simulink model "cleanmodel"  (R2024a)
settings: Solver=VariableStepAuto  StartTime=0.0  StopTime=50  RelTol=1e-3
values from neighbouring files (symbols this model uses):
  b = 1    [Hydrone_model_code.m]
  L = 1.16    [Hydrone_model_code.m]
  r = 1    [Hydrone_model_code.m]
  w = .7    (= 0.7)    [Hydrone_model_code.m]
  WGS1984 = [ 0 0 0; 10 0 0; 10 10 0; 11 20 0; 20 20 0]    [Hydrone_model_code.m]    (also in coverageroi.m = WGS1984(1:size(WGS1984,1)-1,:))
libraries: slpidlib x2, shared6dof x1, robotcorelib x1, uavutilslib x1, uavalgslib x1
settings Model: PacingRate=18  Creator=awolek  LastModifiedBy=alexn
settings RTWCC: GPUComputeCapability=3.5

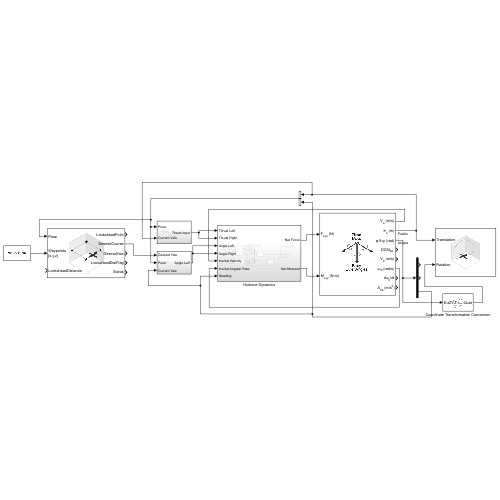
[thumbnail: Simulink's stored preview of the top-level diagram]
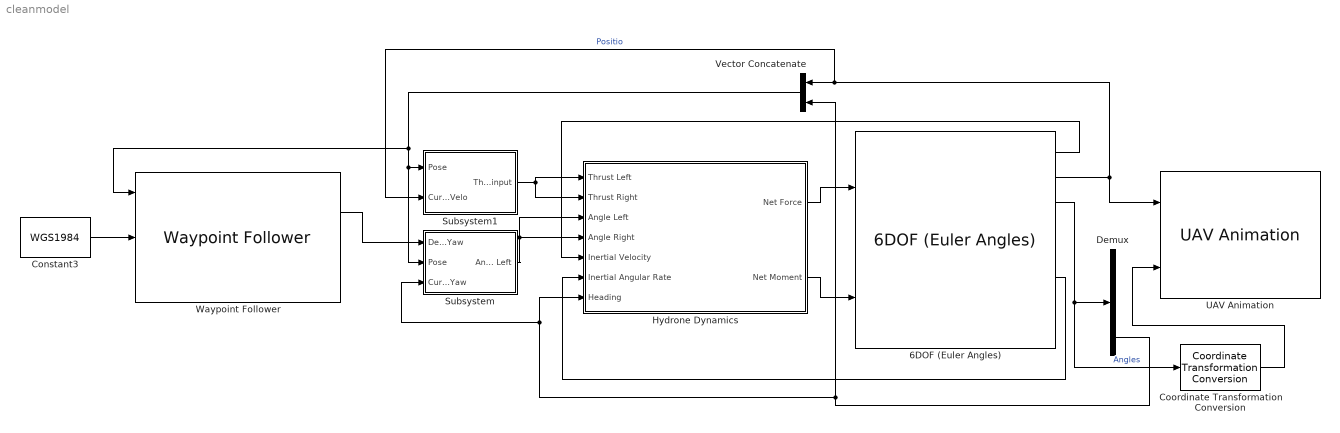
== system cleanmodel ==
  6DOF (Euler Angles) : shared6dof/6DOF (Euler Angles)  units=Metric (MKS)  mtype=Fixed  rep=Euler Angles  xme_0=[0 0 0]  Vm_0=[0 0 0]  eul_0=[0 0 0]  pm_0=[0 0 0]  mass_0=m  mass_e=0.5  mass_f=2.0  inertia=i  inertia_e=eye(3)  inertia_f=2*eye(3)  k_quat=1.0  vre_flag=on  abi_flag=off  aMode=0  xme_statename=''  Vm_statename=''  eul_statename=''  quat_statename=''  pm_statename=''  mass_statename=''
  Constant3 : Constant  Value=WGS1984
  Coordinate Transformation Conversion : robotcorelib/Coordinate Transformation Conversion  InputRepresentation=Euler Angles  InputEulerSequence=ZYZ  ShowTrVecInputPort=on  OutputRepresentation=Quaternion  OutputEulerSequence=ZYX  ShowTrVecOutputPort=on  SimulateUsing=Interpreted execution
      settings: LibrarySourceBlock=uavutilslib/Coordinate Transformation Conversion
  Demux : Demux  Outputs=3
  Hydrone Dynamics : Subsystem
  Subsystem : Subsystem
  Subsystem1 : Subsystem
  UAV Animation : uavutilslib/UAV Animation  UAVType=FixedWing  UAVSize=1  InertialZDirection=Down  SampleTime=-1
  Vector Concatenate : Concatenate
  Waypoint Follower : uavalgslib/Waypoint Follower  UAVType=fixed-wing  StartFrom=first  TransitionRadiusSource=internal  TransitionRadius=1  MinLookaheadDistance=1  YawInput=off  ShowCrossTrackErrorOutput=off  ShowStatusOutput=on  SimulateUsing=Interpreted execution
  wires:
  6DOF (Euler Angles)/2 -> UAV Animation/1, Subsystem1/2(Current Velo), Vector Concatenate/1  "Positio"
  Hydrone Dynamics/1(Net Force) -> 6DOF (Euler Angles)/1
  Hydrone Dynamics/2(Net Moment) -> 6DOF (Euler Angles)/2
  6DOF (Euler Angles)/3 -> Coordinate Transformation Conversion/1, Demux/1  "Angles"
  6DOF (Euler Angles)/6 -> Hydrone Dynamics/6(Inertial Angular Rate)
  Coordinate Transformation Conversion/1 -> UAV Animation/2
  Constant3/1 -> Waypoint Follower/2
  Vector Concatenate/1 -> Subsystem/2(Pose), Subsystem1/1(Pose), Waypoint Follower/1
  6DOF (Euler Angles)/1 -> Hydrone Dynamics/5(Inertial Velocity)
  Waypoint Follower/2 -> Subsystem/1(Desired Yaw)
  Subsystem/1(Angle Left) -> Hydrone Dynamics/3(Angle Left), Hydrone Dynamics/4(Angle Right)
  Demux/3 -> Subsystem/3(Current Yaw), Hydrone Dynamics/7(Heading), Vector Concatenate/2
  Subsystem1/1(Thrust input) -> Hydrone Dynamics/1(Thrust Left), Hydrone Dynamics/2(Thrust Right)

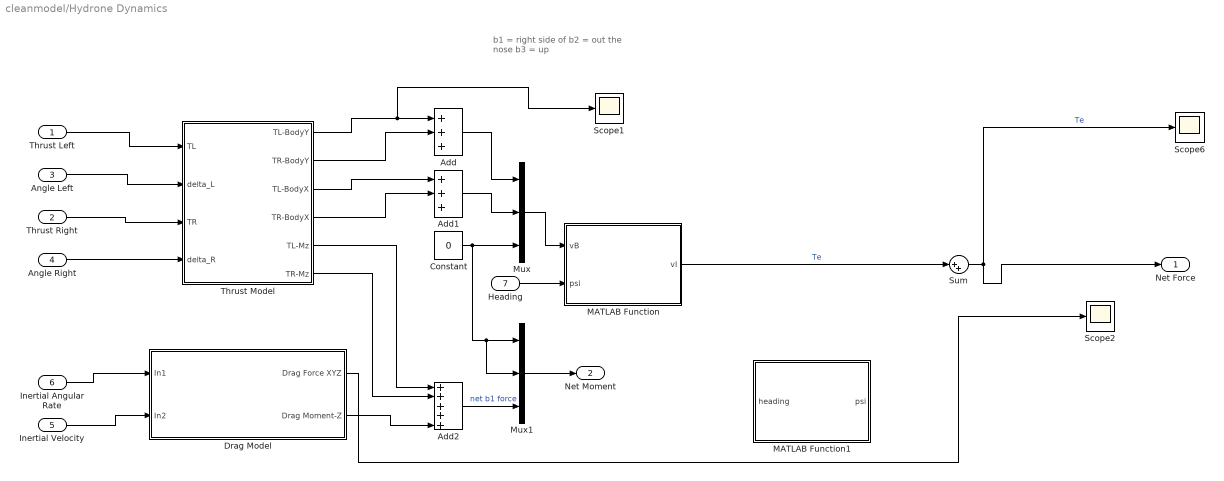
== system cleanmodel/Hydrone Dynamics ==
  note: b1 = right side of
      | b2 = out the nose
      | b3 = up
  Thrust Left : Inport
  Thrust Right : Inport  Port=2
  Angle Left : Inport  Port=3
  Angle Right : Inport  Port=4
  Inertial Velocity : Inport  Port=5
  Inertial Angular Rate : Inport  Port=6
  Heading : Inport  Port=7
  Add : Sum  Inputs=+++
  Add1 : Sum  Inputs=+++
  Add2 : Sum  Inputs=+++++
  Constant : Constant  Value=0
  Drag Model : Subsystem
  MATLAB Function : MATLAB Function  TreatAsAtomicUnit=on
  MATLAB Function1 : MATLAB Function  TreatAsAtomicUnit=on
  Mux : Mux  Inputs=3
  Mux1 : Mux  Inputs=3
  Scope1 : Scope
  Scope2 : Scope
  Scope6 : Scope
  Sum : Sum  Inputs=|++
  Thrust Model : Subsystem
  Net Force : Outport
  Net Moment : Outport  Port=2
  wires:
  Add2/1 -> Mux1/3  "net b1 force"
  Constant/1 -> Mux/3, Mux1/2, Mux1/1
  Drag Model/2(Drag Moment-Z) -> Add2/5
  Mux1/1 -> Net Moment/1
  Thrust Right/1 -> Thrust Model/3(TR)
  Angle Right/1 -> Thrust Model/4(delta_R)
  Inertial Angular Rate/1 -> Drag Model/1(In1)
  Thrust Model/6(TR-Mz) -> Add2/2
  Thrust Model/1(TL-BodyY) -> Scope1/1, Add/1
  Thrust Model/2(TR-BodyY) -> Add/2
  Inertial Velocity/1 -> Drag Model/2(In2)
  Thrust Model/3(TL-BodyX) -> Add1/1
  Angle Left/1 -> Thrust Model/2(delta_L)
  Thrust Model/5(TL-Mz) -> Add2/1
  Thrust Left/1 -> Thrust Model/1(TL)
  Thrust Model/4(TR-BodyX) -> Add1/2
  Add/1 -> Mux/1
  Add1/1 -> Mux/2
  Sum/1 -> Net Force/1, Scope6/1  "Te"
  Heading/1 -> MATLAB Function/2(psi)
  MATLAB Function/1(vI) -> Sum/1  "Te"
  Drag Model/1(Drag Force XYZ) -> Scope2/1
  Mux/1 -> MATLAB Function/1(vB)

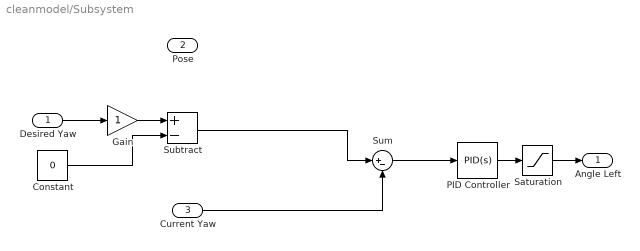
== system cleanmodel/Subsystem ==
  Desired Yaw : Inport
  Pose : Inport  Port=2
  Current Yaw : Inport  Port=3
  Constant : Constant  Value=0
  Gain : Gain
  PID Controller : slpidlib/PID Controller  Controller=PID  Form=Parallel  TimeDomain=Continuous-time  UseExternalTs=off  SampleTime=-1  IntegratorMethod=Forward Euler  FilterMethod=Forward Euler  ControllerParametersSource=internal  P=1  I=.01  UseKiTs=off  D=.001  UseExternalDerivativeSource=off  N=100  UseFilter=on  TunerSelectOption=Transfer Function Based (PID Tuner App)  InitialConditionSource=internal  InitialConditionForIntegrator=0  InitialConditionForFilter=0  DifferentiatorICPrevScaledInput=0  ExternalReset=none  TrackingMode=off  Kt=1  LimitOutput=off  SatLimitsSource=internal  UpperSaturationLimit=inf  LowerSaturationLimit=-inf  LinearizeAsGain=on  AntiWindupMode=none  Kb=1  LimitIntegrator=off  UpperIntegratorSaturationLimit=inf  LowerIntegratorSaturationLimit=-inf  POutMin=[]  POutMax=[]  IOutMin=[]  IOutMax=[]  DOutMin=[]  DOutMax=[]  NOutMin=[]  NOutMax=[]  SumOutMin=[]  SumOutMax=[]  SaturationOutMin=[]  SaturationOutMax=[]  PParamMin=[]  PParamMax=[]  IParamMin=[]  IParamMax=[]  DParamMin=[]  DParamMax=[]  NParamMin=[]  NParamMax=[]  KbParamMin=[]  KbParamMax=[]  KtParamMin=[]  KtParamMax=[]  KbOutMin=[]  KbOutMax=[]  KtOutMin=[]  KtOutMax=[]  IntegratorOutMin=[]  IntegratorOutMax=[]  FilterOutMin=[]  FilterOutMax=[]  SumI1OutMin=[]  SumI1OutMax=[]  SumI2OutMin=[]  SumI2OutMax=[]  SumI3OutMin=[]  SumI3OutMax=[]  SumI4OutMin=[]  SumI4OutMax=[]  SumDOutMin=[]  SumDOutMax=[]  DifferentiatorOutMin=[]  DifferentiatorOutMax=[]  FilterDiffOutCoefMin=[]  FilterDiffOutCoefMax=[]  ReciprocalOutMin=[]  ReciprocalOutMax=[]  SumDenOutMin=[]  SumDenOutMax=[]  SumNumOutMin=[]  SumNumOutMax=[]  DivideOutMin=[]  DivideOutMax=[]  UdiffTsProdOutMin=[]  UdiffTsProdOutMax=[]  NTsProdOutMin=[]  NTsProdOutMax=[]  UintegralTsProdOutMin=[]  UintegralTsProdOutMax=[]  UngainTsProdOutMin=[]  UngainTsProdOutMax=[]  ClampingZeroOutDataTypeStr=Inherit: Inherit via back propagation  ClampingZeroOutMin=[]  ClampingZeroOutMax=[]  FilterDenConstantOutDataTypeStr=Inherit: Inherit via back propagation  FilterDenConstantOutMin=[]  FilterDenConstantOutMax=[]  PCopyOutDataTypeStr=Inherit: Inherit via back propagation  PCopyOutMin=[]  PCopyOutMax=[]  NCopyOutDataTypeStr=Inherit: Inherit via back propagation  NCopyOutMin=[]  NCopyOutMax=[]  IntegratorContinuousStateAttributes=''  IntegratorStateMustResolveToSignalObject=off  IntegratorRTWStateStorageClass=Auto  FilterContinuousStateAttributes=''  FilterStateMustResolveToSignalObject=off  FilterRTWStateStorageClass=Auto  ParallelPVariant=InternalParameters  IdealPVariant=Disabled  IVariant=InternalParameters  DVariant=InternalParameters  IntegratorVariant=Continuous  SatVariant=Disabled  AWVariant=Passthrough  PCopyVariant=Disabled  TRVariant=Disabled  FdbkBlocksVariant=Forward  IdealPFdbkVariant=Disabled  SatFdbkVariant=Disabled  DerivativeFilterVariant=ContFilter  NVariant=InternalParameters  NCopyVariant=Disabled  FilterICVariant=InternalICsFilter  IntegratorICVariant=InternalICs  ExternalResetVariant=Disabled  TRSumVariant=Passthrough  SumFdbkVariant=Disabled  SumVariant=Sum_PID  TsampFilterVariant=InternalTs  TsampNgainVariant=Passthrough  TsampIntegralVariant=Disabled_SignalSpec  ExternalSaturationOutDataTypeStr=Inherit: Same as second input  DerivativeSourceVariant=ErrorSignal
  Saturation : Saturate  UpperLimit=0.78  LowerLimit=-0.78
  Subtract : Sum  Inputs=+-
  Sum : Sum  Inputs=|+-
  Angle Left : Outport
  wires:
  PID Controller/1 -> Saturation/1
  Sum/1 -> PID Controller/1
  Current Yaw/1 -> Sum/2
  Desired Yaw/1 -> Gain/1
  Gain/1 -> Subtract/1
  Constant/1 -> Subtract/2
  Subtract/1 -> Sum/1
  Saturation/1 -> Angle Left/1

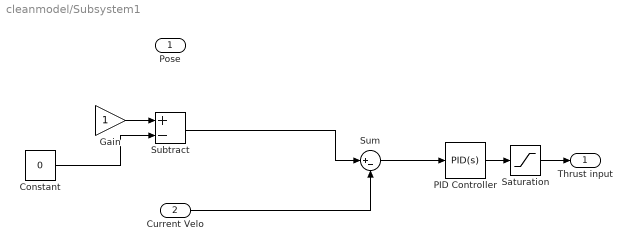
== system cleanmodel/Subsystem1 ==
  Pose : Inport
  Current Velo : Inport  Port=2
  Constant : Constant  Value=0
  Gain : Gain
  PID Controller : slpidlib/PID Controller  Controller=PID  Form=Parallel  TimeDomain=Continuous-time  UseExternalTs=off  SampleTime=-1  IntegratorMethod=Forward Euler  FilterMethod=Forward Euler  ControllerParametersSource=internal  P=1  I=.01  UseKiTs=off  D=.001  UseExternalDerivativeSource=off  N=100  UseFilter=on  TunerSelectOption=Transfer Function Based (PID Tuner App)  InitialConditionSource=internal  InitialConditionForIntegrator=0  InitialConditionForFilter=0  DifferentiatorICPrevScaledInput=0  ExternalReset=none  TrackingMode=off  Kt=1  LimitOutput=off  SatLimitsSource=internal  UpperSaturationLimit=inf  LowerSaturationLimit=-inf  LinearizeAsGain=on  AntiWindupMode=none  Kb=1  LimitIntegrator=off  UpperIntegratorSaturationLimit=inf  LowerIntegratorSaturationLimit=-inf  POutMin=[]  POutMax=[]  IOutMin=[]  IOutMax=[]  DOutMin=[]  DOutMax=[]  NOutMin=[]  NOutMax=[]  SumOutMin=[]  SumOutMax=[]  SaturationOutMin=[]  SaturationOutMax=[]  PParamMin=[]  PParamMax=[]  IParamMin=[]  IParamMax=[]  DParamMin=[]  DParamMax=[]  NParamMin=[]  NParamMax=[]  KbParamMin=[]  KbParamMax=[]  KtParamMin=[]  KtParamMax=[]  KbOutMin=[]  KbOutMax=[]  KtOutMin=[]  KtOutMax=[]  IntegratorOutMin=[]  IntegratorOutMax=[]  FilterOutMin=[]  FilterOutMax=[]  SumI1OutMin=[]  SumI1OutMax=[]  SumI2OutMin=[]  SumI2OutMax=[]  SumI3OutMin=[]  SumI3OutMax=[]  SumI4OutMin=[]  SumI4OutMax=[]  SumDOutMin=[]  SumDOutMax=[]  DifferentiatorOutMin=[]  DifferentiatorOutMax=[]  FilterDiffOutCoefMin=[]  FilterDiffOutCoefMax=[]  ReciprocalOutMin=[]  ReciprocalOutMax=[]  SumDenOutMin=[]  SumDenOutMax=[]  SumNumOutMin=[]  SumNumOutMax=[]  DivideOutMin=[]  DivideOutMax=[]  UdiffTsProdOutMin=[]  UdiffTsProdOutMax=[]  NTsProdOutMin=[]  NTsProdOutMax=[]  UintegralTsProdOutMin=[]  UintegralTsProdOutMax=[]  UngainTsProdOutMin=[]  UngainTsProdOutMax=[]  ClampingZeroOutDataTypeStr=Inherit: Inherit via back propagation  ClampingZeroOutMin=[]  ClampingZeroOutMax=[]  FilterDenConstantOutDataTypeStr=Inherit: Inherit via back propagation  FilterDenConstantOutMin=[]  FilterDenConstantOutMax=[]  PCopyOutDataTypeStr=Inherit: Inherit via back propagation  PCopyOutMin=[]  PCopyOutMax=[]  NCopyOutDataTypeStr=Inherit: Inherit via back propagation  NCopyOutMin=[]  NCopyOutMax=[]  IntegratorContinuousStateAttributes=''  IntegratorStateMustResolveToSignalObject=off  IntegratorRTWStateStorageClass=Auto  FilterContinuousStateAttributes=''  FilterStateMustResolveToSignalObject=off  FilterRTWStateStorageClass=Auto  ParallelPVariant=InternalParameters  IdealPVariant=Disabled  IVariant=InternalParameters  DVariant=InternalParameters  IntegratorVariant=Continuous  SatVariant=Disabled  AWVariant=Passthrough  PCopyVariant=Disabled  TRVariant=Disabled  FdbkBlocksVariant=Forward  IdealPFdbkVariant=Disabled  SatFdbkVariant=Disabled  DerivativeFilterVariant=ContFilter  NVariant=InternalParameters  NCopyVariant=Disabled  FilterICVariant=InternalICsFilter  IntegratorICVariant=InternalICs  ExternalResetVariant=Disabled  TRSumVariant=Passthrough  SumFdbkVariant=Disabled  SumVariant=Sum_PID  TsampFilterVariant=InternalTs  TsampNgainVariant=Passthrough  TsampIntegralVariant=Disabled_SignalSpec  ExternalSaturationOutDataTypeStr=Inherit: Same as second input  DerivativeSourceVariant=ErrorSignal
  Saturation : Saturate  UpperLimit=0.78  LowerLimit=-0.78
  Subtract : Sum  Inputs=+-
  Sum : Sum  Inputs=|+-
  Thrust input : Outport
  wires:
  PID Controller/1 -> Saturation/1
  Sum/1 -> PID Controller/1
  Current Velo/1 -> Sum/2
  ? -> Gain/1
  Gain/1 -> Subtract/1
  Constant/1 -> Subtract/2
  Subtract/1 -> Sum/1
  Saturation/1 -> Thrust input/1

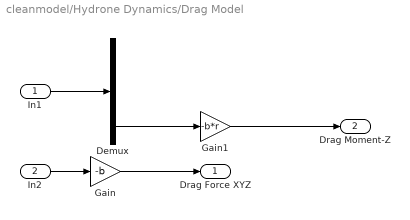
== system cleanmodel/Hydrone Dynamics/Drag Model ==
  In1 : Inport
  In2 : Inport  Port=2
  Demux : Demux  Outputs=3
  Gain : Gain  Gain=-b
  Gain1 : Gain  Gain=-b*r
  Drag Force XYZ : Outport
  Drag Moment-Z : Outport  Port=2
  wires:
  Gain1/1 -> Drag Moment-Z/1
  Gain/1 -> Drag Force XYZ/1
  In2/1 -> Gain/1
  In1/1 -> Demux/1
  Demux/3 -> Gain1/1

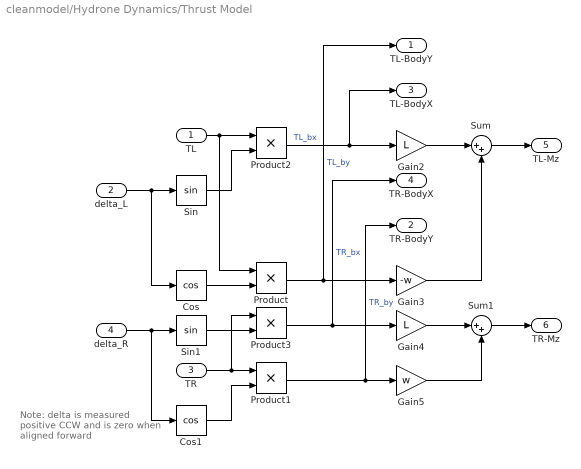
== system cleanmodel/Hydrone Dynamics/Thrust Model ==
  note: Note: delta is measured
      | positive CCW and is
      | zero when aligned
      | forward
  TL : Inport
  delta_L : Inport  Port=2
  TR : Inport  Port=3
  delta_R : Inport  Port=4
  Cos : Trigonometry  Operator=cos
  Cos1 : Trigonometry  Operator=cos
  Gain2 : Gain  Gain=L
  Gain3 : Gain  Gain=-w
  Gain4 : Gain  Gain=L
  Gain5 : Gain  Gain=w
  Product{,1..3} (4 alike) : Product
  Sin : Trigonometry
  Sin1 : Trigonometry
  Sum : Sum  Inputs=|++
  Sum1 : Sum  Inputs=|++
  TL-BodyY : Outport
  TR-BodyY : Outport  Port=2
  TL-BodyX : Outport  Port=3
  TR-BodyX : Outport  Port=4
  TL-Mz : Outport  Port=5
  TR-Mz : Outport  Port=6
  wires:
  Sum/1 -> TL-Mz/1
  Gain5/1 -> Sum1/2
  Gain4/1 -> Sum1/1
  delta_L/1 -> Cos/1, Sin/1
  Cos1/1 -> Product1/2
  delta_R/1 -> Cos1/1, Sin1/1
  TR/1 -> Product3/1, Product1/1
  TL/1 -> Product/1, Product2/1
  Sin1/1 -> Product3/2
  Sin/1 -> Product2/2
  Sum1/1 -> TR-Mz/1
  Gain3/1 -> Sum/2
  Product/1 -> TL-BodyY/1, Gain3/1  "TL_by"
  Cos/1 -> Product/2
  Product2/1 -> TL-BodyX/1, Gain2/1  "TL_bx"
  Product3/1 -> Gain4/1, TR-BodyX/1  "TR_bx"
  Product1/1 -> TR-BodyY/1, Gain5/1  "TR_by"
  Gain2/1 -> Sum/1

== matlab function cleanmodel/Hydrone Dynamics/MATLAB Function ==
  data: vB input; vI output; psi input
function vI = R_BtoI(vB, psi)
% R_BtoI=eye(3);
R_BtoI = [cos(psi) -sin(psi) 0;
         sin(psi) cos(psi) 0;
         0         0        1];
vI = R_BtoI*vB;

== matlab function cleanmodel/Hydrone Dynamics/MATLAB Function1 ==
  data: heading input; psi output
function psi = fix(heading)

psi=(heading/2);
